simulink model "nms_model"  (Simulink 7.5)
settings: Solver=ode15s  StartTime=0.0  StopTime=60  FixedStep=1e-3  MaxStep=ts_max  RelTol=1e-3  AbsTol=1e-4
InitFcn:
  | nms_model_MechInit
  | nms_model_ControlInit
values from neighbouring files (symbols this model uses):
  c = 0.05    [muscleParams.m]    (also in nms_model_MechInit.m)
  c_jointstop = 0.3 / (pi/180)    (= 17.1887338539)    [muscleParams.m]    (also in nms_model_MechInit.m)
  D12_F = 0.16    [nms_model_MechInit.m]
  D12_S = L_S    (= 0.5)    [nms_model_MechInit.m]
  D12_T = L_T    (= 0.5)    [nms_model_MechInit.m]
  D13_F = 0.20    (= 0.2)    [nms_model_MechInit.m]
  D1G_F = 0.14    [nms_model_MechInit.m]
  D1G_HAT = 0.35    [nms_model_MechInit.m]
  D1G_S = 0.3    [nms_model_MechInit.m]
  D1G_T = 0.3    [nms_model_MechInit.m]
  DeltaThRef = 5e-3    (= 0.005)    [nms_model_MechInit.m]
  eref = 0.04    [muscleParams.m]    (also in nms_model_MechInit.m)
  FmaxGAS = 1500    [nms_model_MechInit.m]
  FmaxGLU = 1500    [nms_model_MechInit.m]
  FmaxHAM = 3000    [nms_model_MechInit.m]
  FmaxHFL = 2000    [nms_model_MechInit.m]
  FmaxSOL = 4000    [nms_model_MechInit.m]
  FmaxTA = 800    [nms_model_MechInit.m]
  FmaxVAS = 300    [muscleParams.m]    (also in nms_model_MechInit.m = 6000)
  GainDeltaTheta = 2 /100*180/pi    (= 1.14591559026)    [nms_model_ControlInit.m]
  GainGAS = 1.1/FmaxGAS    [nms_model_ControlInit.m]
  GainGLU = 0.5/FmaxGLU    [nms_model_ControlInit.m]
  GainHAM = 0.65/FmaxHAM    [nms_model_ControlInit.m]
  GainHAMHFL = 4    [nms_model_ControlInit.m]
  GainHFL = 0.5    [nms_model_ControlInit.m]
  GainKneOverExt = 2    [nms_model_ControlInit.m]
  GainSOL = 1.2/FmaxSOL    [nms_model_ControlInit.m]
  GainSOLTA = 0.4/FmaxSOL    [nms_model_ControlInit.m]
  GainTA = 1.1    [nms_model_ControlInit.m]
  GainVAS = 1.2/FmaxVAS    [nms_model_ControlInit.m]
  In_F = 0.005    [nms_model_MechInit.m]
  In_HAT = 3    [nms_model_MechInit.m]
  In_S = 0.05    [nms_model_MechInit.m]
  In_T = 0.15    [nms_model_MechInit.m]
  K = 5    [muscleParams.m]    (also in nms_model_MechInit.m)
  k_gx = (2*(m_F+m_S+m_T)+m_HAT)*g/0.1    (= 7848)    [nms_model_MechInit.m]
  k_gy = (2*(m_F+m_S+m_T)+m_HAT)*g/0.01    (= 78480)    [nms_model_MechInit.m]
  k_pressure = m_HAT * 9.81 / DeltaThRef    (= 104967)    [nms_model_MechInit.m]
  K_swing = 0.25    [nms_model_ControlInit.m]
  KneePh23Offset = 170*pi/180    (= 2.96705972839)    [nms_model_ControlInit.m]
  LceOffsetHAM = 0.85    [nms_model_ControlInit.m]
  LceOffsetHFL = 0.65    [nms_model_ControlInit.m]
  LceOffsetTA = 1-0.5*w    [nms_model_ControlInit.m]
  LongDelay = 0.020    (= 0.02)    [nms_model_ControlInit.m]
  loptGAS = 0.05    [nms_model_MechInit.m]
  loptGLU = 0.11    [nms_model_MechInit.m]
  loptHAM = 0.10    (= 0.1)    [nms_model_MechInit.m]
  loptHFL = 0.11    [nms_model_MechInit.m]
  loptSOL = 0.04    [nms_model_MechInit.m]
  loptTA = 0.06    [nms_model_MechInit.m]
  loptVAS = 0.13    [muscleParams.m]    (also in nms_model_MechInit.m = 0.08)
  lslackGAS = 0.40    (= 0.4)    [nms_model_MechInit.m]
  lslackGLU = 0.13    [nms_model_MechInit.m]
  lslackHAM = 0.31    [nms_model_MechInit.m]
  lslackHFL = 0.10    (= 0.1)    [nms_model_MechInit.m]
  lslackSOL = 0.26    [nms_model_MechInit.m]
  lslackTA = 0.24    [nms_model_MechInit.m]
  lslackVAS = 0.23    [muscleParams.m]    (also in nms_model_MechInit.m)
  m_F = 1.25    [nms_model_MechInit.m]
  m_HAT = 53.5    [nms_model_MechInit.m]
  m_S = 3.5    [nms_model_MechInit.m]
  m_T = 8.5    [nms_model_MechInit.m]
  MidDelay = 0.010    (= 0.01)    [nms_model_ControlInit.m]
  mu_slide = 0.8    [nms_model_MechInit.m]
  mu_stick = 0.9    [nms_model_MechInit.m]
  N = 1.5    [muscleParams.m]    (also in nms_model_MechInit.m)
  phi12_LowLimit = 70*pi/180    (= 1.2217304764)    [nms_model_MechInit.m]
  phi12_UpLimit = 180*pi/180    (= 3.14159265359)    [muscleParams.m]    (also in nms_model_MechInit.m = 2.26892802759)
  phi23_UpLimit = 159*pi/180    (= 2.77507351067)    [muscleParams.m]    (also in nms_model_MechInit.m = 3.05432619099)
  phi34_UpLimit = 230*pi/180    (= 4.01425727959)    [nms_model_MechInit.m]
  phimaxGASa = 110*pi/180    (= 1.91986217719)    [nms_model_MechInit.m]
  phimaxGASk = 140*pi/180    (= 2.44346095279)    [nms_model_MechInit.m]
  phimaxHAMk = 180*pi/180    (= 3.14159265359)    [nms_model_MechInit.m]
  phimaxSOL = 110*pi/180    (= 1.91986217719)    [nms_model_MechInit.m]
  phimaxTA = 80*pi/180    (= 1.3962634016)    [nms_model_MechInit.m]
  phimaxVAS = 90*pi/180    (= 1.57079632679)    [muscleParams.m]    (also in nms_model_MechInit.m = 2.87979326579)
  phirefGASa = 80*pi/180    (= 1.3962634016)    [nms_model_MechInit.m]
  phirefGASk = 165*pi/180    (= 2.87979326579)    [nms_model_MechInit.m]
  phirefGLU = 150*pi/180    (= 2.61799387799)    [nms_model_MechInit.m]
  phirefHAMh = 155*pi/180    (= 2.70526034059)    [nms_model_MechInit.m]
  phirefHAMk = 180*pi/180    (= 3.14159265359)    [nms_model_MechInit.m]
  phirefHFL = 180*pi/180    (= 3.14159265359)    [nms_model_MechInit.m]
  phirefSOL = 80*pi/180    (= 1.3962634016)    [nms_model_MechInit.m]
  phirefTA = 110*pi/180    (= 1.91986217719)    [nms_model_MechInit.m]
  phirefVAS = 60*pi/180    (= 1.0471975512)    [muscleParams.m]    (also in nms_model_MechInit.m = 2.18166156499)
  PosGainGG = 1/(30*pi/180)    (= 1.9098593171)    [nms_model_ControlInit.m]
  PreStimGAS = 0.01    [nms_model_ControlInit.m]
  PreStimGG = 0.05    [nms_model_ControlInit.m]
  PreStimGLU = 0.01    [nms_model_ControlInit.m]
  PreStimHAM = 0.01    [nms_model_ControlInit.m]
  PreStimHFL = 0.01    [nms_model_ControlInit.m]
  PreStimSOL = 0.01    [nms_model_ControlInit.m]
  PreStimTA = 0.01    [nms_model_ControlInit.m]
  PreStimVAS = 0.08    [nms_model_ControlInit.m]
  rGASa = 0.05    [nms_model_MechInit.m]
  rGASk = 0.05    [nms_model_MechInit.m]
  rGLU = 0.10    (= 0.1)    [nms_model_MechInit.m]
  rHAMh = 0.08    [nms_model_MechInit.m]
  rHAMk = 0.05    [nms_model_MechInit.m]
  rHFL = 0.10    (= 0.1)    [nms_model_MechInit.m]
  rhoGASa = 0.7    [nms_model_MechInit.m]
  rhoGASk = 0.7    [nms_model_MechInit.m]
  rhoGLU = 0.5    [nms_model_MechInit.m]
  rhoHAMh = 0.7    [nms_model_MechInit.m]
  rhoHAMk = 0.7    [nms_model_MechInit.m]
  rhoHFL = 0.5    [nms_model_MechInit.m]
  rhoSOL = 0.5    [nms_model_MechInit.m]
  rhoTA = 0.7    [nms_model_MechInit.m]
  rhoVAS = 3    [muscleParams.m]    (also in nms_model_MechInit.m = 0.7)
  rSOL = 0.05    [nms_model_MechInit.m]
  rTA = 0.04    [nms_model_MechInit.m]
  rVAS = 0.03    [muscleParams.m]    (also in nms_model_MechInit.m = 0.06)
  s = orProblemSendCommand(['LoadIKFastSolver robot Translation3D'],probid)    [init.m]
  ShortDelay = 0.005    [nms_model_ControlInit.m]
  SpeedGainGG = 0.2    [nms_model_ControlInit.m]
  tau = 0.01    [muscleParams.m]    (also in nms_model_MechInit.m)
  Theta0 = 6*pi/180    (= 0.10471975512)    [nms_model_ControlInit.m]
  ThPos = 4/5    (= 0.8)    [nms_model_MechInit.m]
  v_gx_max = 0.03    [nms_model_MechInit.m]
  v_gy_max = 0.03    [nms_model_MechInit.m]
  ... (+11 more)
undefined symbols (not defined in the file or in its folder): sgn
libraries: mblibv1 x60, simulink x22, simulink_extras x20
(part 9 of 9)

== system nms_model/Body Mechanics Layer/Left Ball Contact/Ground Friction Model/X-Axis Kinetic Friction Model ==
  note: Kinetic Friction Model
  note: Footpoint Determiner
  note: Sliding Limit Detector
  pos [m] : Inport  OutDataType=sfix(16)  OutScaling=2^0
  vel [m/s] : Inport  Port=2  OutDataType=sfix(16)  OutScaling=2^0
  F_Normal [N] : Inport  Port=3  OutDataType=sfix(16)  OutScaling=2^0
  Enable : EnablePort  StatesWhenEnabling=reset  ZeroCross=off
  Abs : Abs
  Constant : Constant  Value=vLimit  OutDataType=sfix(16)  OutScaling=2^0
  FixPt Relational Operator : RelationalOperator  Operator=>  LogicOutDataTypeMode=boolean  OutDataTypeStr=boolean  ZeroCross=off
  Memory : Memory
  Negative : simulink/Logic and Bit Operations/Compare To Zero  SystemSampleTime=-1  relop=<  LogicOutDataTypeMode=boolean
  Product : Product  OutDataType=sfix(16)  OutScaling=2^0  RndMeth=Zero
  Sign1 : Signum
  Sum : Sum  Inputs=|+-  OutDataType=sfix(16)  OutScaling=2^0
  reverse : Gain  Gain=-1  ParameterDataType=sfix(16)  ParameterScaling=2^0  OutDataType=sfix(16)  OutScaling=2^0
  sliding friction coefficient : Gain  Gain=mu_slide  ParameterDataType=sfix(16)  ParameterScaling=2^0  OutDataType=sfix(16)  OutScaling=2^0
  posFP [m] : Outport  OutDataType=sfix(16)  OutScaling=2^0  InitialOutput=0
      settings: AttributesFormatString=initial = '%<InitialOutput>'\nwhen disabled = '%<OutputWhenDisabled>'
  Stiction! : Outport  Port=2  OutDataType=sfix(16)  OutScaling=2^0  OutputWhenDisabled=reset  InitialOutput=0
      settings: AttributesFormatString=initial = '%<InitialOutput>'\nwhen disabled = '%<OutputWhenDisabled>'
  F_Slide [N] : Outport  Port=3  OutDataType=sfix(16)  OutScaling=2^0  OutputWhenDisabled=reset  InitialOutput=0
      settings: AttributesFormatString=initial = '%<InitialOutput>'\nwhen disabled = '%<OutputWhenDisabled>'
  wires:
  reverse/1 -> Product/1
  F_Normal [N]/1 -> sliding friction coefficient/1
  vel [m/s]/1 -> Sign1/1, Abs/1
  pos [m]/1 -> posFP [m]/1
  Product/1 -> F_Slide [N]/1
  sliding friction coefficient/1 -> Product/2
  Sign1/1 -> reverse/1
  FixPt Relational Operator/1 -> Stiction!/1
  Memory/1 -> FixPt Relational Operator/2
  Negative/1 -> FixPt Relational Operator/1, Memory/1
  Abs/1 -> Sum/1
  Sum/1 -> Negative/1
  Constant/1 -> Sum/2

== system nms_model/Body Mechanics Layer/Left Ball Contact/Ground Friction Model/X-Axis Static Friction Model ==
  note: Stiction Limit Detector
  note: Static Friction Model
  note: Zero multiplication prevents
      | horizontal friction model from
      | oscillating between static and kinetic
      | friction when the vertical force is zero but
      | the ground level is not yet reached
      | in the upward motion
  F_Normal [N] : Inport  OutDataType=sfix(16)  OutScaling=2^0
  pos [m] : Inport  Port=2  OutDataType=sfix(16)  OutScaling=2^0
  vel [m/s] : Inport  Port=3  OutDataType=sfix(16)  OutScaling=2^0
  posFP [m] : Inport  Port=4  OutDataType=sfix(16)  OutScaling=2^0
  Enable : EnablePort  StatesWhenEnabling=reset  ZeroCross=off
  Abs : Abs
  Abs. : Abs
  Check Vertical Friction : Product  OutDataType=sfix(16)  OutScaling=2^0  RndMeth=Zero
  FixPt Relational Operator : RelationalOperator  Operator=>  LogicOutDataTypeMode=boolean  OutDataTypeStr=boolean  ZeroCross=off
  Gain3 : Gain  Gain=k_gx  ParameterDataType=sfix(16)  ParameterScaling=2^0  OutDataType=sfix(16)  OutScaling=2^0
  Gain4 : Gain  Gain=1/v_gx_max  ParameterDataType=sfix(16)  ParameterScaling=2^0  OutDataType=sfix(16)  OutScaling=2^0
  Memory : Memory
  Mux1 : Mux  Inputs=2
  Positive : simulink/Logic and Bit Operations/Compare To Zero  SystemSampleTime=-1  relop=>  LogicOutDataTypeMode=boolean
  Positive1 : simulink/Logic and Bit Operations/Compare To Zero  SystemSampleTime=-1  relop=>  LogicOutDataTypeMode=boolean
  Sum : Sum  Inputs=-+  OutDataType=sfix(16)  OutScaling=2^0
  Sum2 : Sum  Inputs=-+|  OutDataType=sfix(16)  OutScaling=2^0
  X-Axis Stiction Force : Fcn  Expr=-u(1) * (1+sgn(u(1))*u(2))
  stiction limit force : Gain  Gain=mu_stick  ParameterDataType=sfix(16)  ParameterScaling=2^0  OutDataType=sfix(16)  OutScaling=2^0
  F_Stick [N] : Outport  OutDataType=sfix(16)  OutScaling=2^0  OutputWhenDisabled=reset  InitialOutput=0
      settings: AttributesFormatString=when disabled: %<OutputWhenDisabled>\ninitial: %<InitialOutput>
  Sliding! : Outport  Port=2  OutDataType=sfix(16)  OutScaling=2^0  OutputWhenDisabled=reset  InitialOutput=0
      settings: AttributesFormatString=when disabled: %<OutputWhenDisabled>\ninitial: %<InitialOutput>
  wires:
  F_Normal [N]/1 -> stiction limit force/1, Positive1/1
  Sum2/1 -> Gain3/1  "dx"
  pos [m]/1 -> Sum2/2
  posFP [m]/1 -> Sum2/1
  vel [m/s]/1 -> Gain4/1
  Sum/1 -> Positive/1
  Memory/1 -> FixPt Relational Operator/2
  Positive/1 -> FixPt Relational Operator/1, Memory/1
  Abs./1 -> Sum/2
  Mux1/1 -> X-Axis Stiction Force/1
  Gain3/1 -> Mux1/1
  Gain4/1 -> Mux1/2
  FixPt Relational Operator/1 -> Sliding!/1
  Abs/1 -> Sum/1
  stiction limit force/1 -> Abs/1
  X-Axis Stiction Force/1 -> Check Vertical Friction/1
  Positive1/1 -> Check Vertical Friction/2
  Check Vertical Friction/1 -> F_Stick [N]/1, Abs./1

== system nms_model/Body Mechanics Layer/Left Heel Contact/Ground Friction Model/Friction Switch ==
  note: Static/Kinetic Friction Switch
  Slide! : Inport  OutDataType=sfix(16)  OutScaling=2^0
  Stick! : Inport  Port=2  OutDataType=sfix(16)  OutScaling=2^0
  Memory : Memory
  S-R Flip-Flop : simulink_extras/Flip Flops/S-R Flip-Flop  SystemSampleTime=-1  initial_condition=1
  Terminator : Terminator
  Stiction : Outport  OutDataType=sfix(16)  OutScaling=2^0
  wires:
  Memory/1 -> Stiction/1
  Slide!/1 -> S-R Flip-Flop/2
  Stick!/1 -> S-R Flip-Flop/1
  S-R Flip-Flop/2 -> Terminator/1
  S-R Flip-Flop/1 -> Memory/1

== system nms_model/Body Mechanics Layer/Left Heel Contact/Ground Friction Model/X-Axis Kinetic Friction Model ==
  note: Sliding Limit Detector
  note: Footpoint Determiner
  note: Kinetic Friction Model
  pos [m] : Inport  OutDataType=sfix(16)  OutScaling=2^0
  vel [m/s] : Inport  Port=2  OutDataType=sfix(16)  OutScaling=2^0
  F_Normal [N] : Inport  Port=3  OutDataType=sfix(16)  OutScaling=2^0
  Enable : EnablePort  StatesWhenEnabling=reset  ZeroCross=off
  Abs : Abs
  Constant : Constant  Value=vLimit  OutDataType=sfix(16)  OutScaling=2^0
  FixPt Relational Operator : RelationalOperator  Operator=>  LogicOutDataTypeMode=boolean  OutDataTypeStr=boolean  ZeroCross=off
  Memory : Memory
  Negative : simulink/Logic and Bit Operations/Compare To Zero  SystemSampleTime=-1  relop=<  LogicOutDataTypeMode=boolean
  Product : Product  OutDataType=sfix(16)  OutScaling=2^0  RndMeth=Zero
  Sign1 : Signum
  Sum : Sum  Inputs=|+-  OutDataType=sfix(16)  OutScaling=2^0
  reverse : Gain  Gain=-1  ParameterDataType=sfix(16)  ParameterScaling=2^0  OutDataType=sfix(16)  OutScaling=2^0
  sliding friction coefficient : Gain  Gain=mu_slide  ParameterDataType=sfix(16)  ParameterScaling=2^0  OutDataType=sfix(16)  OutScaling=2^0
  posFP [m] : Outport  OutDataType=sfix(16)  OutScaling=2^0  InitialOutput=0
      settings: AttributesFormatString=initial = '%<InitialOutput>'\nwhen disabled = '%<OutputWhenDisabled>'
  Stiction! : Outport  Port=2  OutDataType=sfix(16)  OutScaling=2^0  OutputWhenDisabled=reset  InitialOutput=0
      settings: AttributesFormatString=initial = '%<InitialOutput>'\nwhen disabled = '%<OutputWhenDisabled>'
  F_Slide [N] : Outport  Port=3  OutDataType=sfix(16)  OutScaling=2^0  OutputWhenDisabled=reset  InitialOutput=0
      settings: AttributesFormatString=initial = '%<InitialOutput>'\nwhen disabled = '%<OutputWhenDisabled>'
  wires:
  Constant/1 -> Sum/2
  Sum/1 -> Negative/1
  Abs/1 -> Sum/1
  Negative/1 -> Memory/1, FixPt Relational Operator/1
  Memory/1 -> FixPt Relational Operator/2
  FixPt Relational Operator/1 -> Stiction!/1
  Sign1/1 -> reverse/1
  sliding friction coefficient/1 -> Product/2
  Product/1 -> F_Slide [N]/1
  pos [m]/1 -> posFP [m]/1
  vel [m/s]/1 -> Abs/1, Sign1/1
  F_Normal [N]/1 -> sliding friction coefficient/1
  reverse/1 -> Product/1

== system nms_model/Body Mechanics Layer/Left Heel Contact/Ground Friction Model/X-Axis Static Friction Model ==
  note: Static Friction Model
  note: Stiction Limit Detector
  note: Zero multiplication prevents
      | horizontal friction model from
      | oscillating between static and kinetic
      | friction when the vertical force is zero but
      | the ground level is not yet reached
      | in the upward motion
  F_Normal [N] : Inport  OutDataType=sfix(16)  OutScaling=2^0
  pos [m] : Inport  Port=2  OutDataType=sfix(16)  OutScaling=2^0
  vel [m/s] : Inport  Port=3  OutDataType=sfix(16)  OutScaling=2^0
  posFP [m] : Inport  Port=4  OutDataType=sfix(16)  OutScaling=2^0
  Enable : EnablePort  StatesWhenEnabling=reset  ZeroCross=off
  Abs : Abs
  Abs. : Abs
  Check Vertical Friction : Product  OutDataType=sfix(16)  OutScaling=2^0  RndMeth=Zero
  FixPt Relational Operator : RelationalOperator  Operator=>  LogicOutDataTypeMode=boolean  OutDataTypeStr=boolean  ZeroCross=off
  Gain3 : Gain  Gain=k_gx  ParameterDataType=sfix(16)  ParameterScaling=2^0  OutDataType=sfix(16)  OutScaling=2^0
  Gain4 : Gain  Gain=1/v_gx_max  ParameterDataType=sfix(16)  ParameterScaling=2^0  OutDataType=sfix(16)  OutScaling=2^0
  Memory : Memory
  Mux1 : Mux  Inputs=2
  Positive : simulink/Logic and Bit Operations/Compare To Zero  SystemSampleTime=-1  relop=>  LogicOutDataTypeMode=boolean
  Positive1 : simulink/Logic and Bit Operations/Compare To Zero  SystemSampleTime=-1  relop=>  LogicOutDataTypeMode=boolean
  Sum : Sum  Inputs=-+  OutDataType=sfix(16)  OutScaling=2^0
  Sum2 : Sum  Inputs=-+|  OutDataType=sfix(16)  OutScaling=2^0
  X-Axis Stiction Force : Fcn  Expr=-u(1) * (1+sgn(u(1))*u(2))
  stiction limit force : Gain  Gain=mu_stick  ParameterDataType=sfix(16)  ParameterScaling=2^0  OutDataType=sfix(16)  OutScaling=2^0
  F_Stick [N] : Outport  OutDataType=sfix(16)  OutScaling=2^0  OutputWhenDisabled=reset  InitialOutput=0
      settings: AttributesFormatString=when disabled: %<OutputWhenDisabled>\ninitial: %<InitialOutput>
  Sliding! : Outport  Port=2  OutDataType=sfix(16)  OutScaling=2^0  OutputWhenDisabled=reset  InitialOutput=0
      settings: AttributesFormatString=when disabled: %<OutputWhenDisabled>\ninitial: %<InitialOutput>
  wires:
  F_Normal [N]/1 -> stiction limit force/1, Positive1/1
  Sum2/1 -> Gain3/1  "dx"
  pos [m]/1 -> Sum2/2
  posFP [m]/1 -> Sum2/1
  vel [m/s]/1 -> Gain4/1
  Sum/1 -> Positive/1
  Memory/1 -> FixPt Relational Operator/2
  Positive/1 -> FixPt Relational Operator/1, Memory/1
  Abs./1 -> Sum/2
  Mux1/1 -> X-Axis Stiction Force/1
  Gain3/1 -> Mux1/1
  Gain4/1 -> Mux1/2
  FixPt Relational Operator/1 -> Sliding!/1
  Abs/1 -> Sum/1
  stiction limit force/1 -> Abs/1
  X-Axis Stiction Force/1 -> Check Vertical Friction/1
  Positive1/1 -> Check Vertical Friction/2
  Check Vertical Friction/1 -> F_Stick [N]/1, Abs./1

== system nms_model/Body Mechanics Layer/Right Ball Contact/Ground Friction Model/Friction Switch ==
  note: Static/Kinetic Friction Switch
  Slide! : Inport  OutDataType=sfix(16)  OutScaling=2^0
  Stick! : Inport  Port=2  OutDataType=sfix(16)  OutScaling=2^0
  Memory : Memory
  S-R Flip-Flop : simulink_extras/Flip Flops/S-R Flip-Flop  SystemSampleTime=-1  initial_condition=1
  Terminator : Terminator
  Stiction : Outport  OutDataType=sfix(16)  OutScaling=2^0
  wires:
  S-R Flip-Flop/1 -> Memory/1
  S-R Flip-Flop/2 -> Terminator/1
  Stick!/1 -> S-R Flip-Flop/1
  Slide!/1 -> S-R Flip-Flop/2
  Memory/1 -> Stiction/1

== system nms_model/Body Mechanics Layer/Right Ball Contact/Ground Friction Model/X-Axis Kinetic Friction Model ==
  note: Kinetic Friction Model
  note: Footpoint Determiner
  note: Sliding Limit Detector
  pos [m] : Inport  OutDataType=sfix(16)  OutScaling=2^0
  vel [m/s] : Inport  Port=2  OutDataType=sfix(16)  OutScaling=2^0
  F_Normal [N] : Inport  Port=3  OutDataType=sfix(16)  OutScaling=2^0
  Enable : EnablePort  StatesWhenEnabling=reset  ZeroCross=off
  Abs : Abs
  Constant : Constant  Value=vLimit  OutDataType=sfix(16)  OutScaling=2^0
  FixPt Relational Operator : RelationalOperator  Operator=>  LogicOutDataTypeMode=boolean  OutDataTypeStr=boolean  ZeroCross=off
  Memory : Memory
  Negative : simulink/Logic and Bit Operations/Compare To Zero  SystemSampleTime=-1  relop=<  LogicOutDataTypeMode=boolean
  Product : Product  OutDataType=sfix(16)  OutScaling=2^0  RndMeth=Zero
  Sign1 : Signum
  Sum : Sum  Inputs=|+-  OutDataType=sfix(16)  OutScaling=2^0
  reverse : Gain  Gain=-1  ParameterDataType=sfix(16)  ParameterScaling=2^0  OutDataType=sfix(16)  OutScaling=2^0
  sliding friction coefficient : Gain  Gain=mu_slide  ParameterDataType=sfix(16)  ParameterScaling=2^0  OutDataType=sfix(16)  OutScaling=2^0
  posFP [m] : Outport  OutDataType=sfix(16)  OutScaling=2^0  InitialOutput=0
      settings: AttributesFormatString=initial = '%<InitialOutput>'\nwhen disabled = '%<OutputWhenDisabled>'
  Stiction! : Outport  Port=2  OutDataType=sfix(16)  OutScaling=2^0  OutputWhenDisabled=reset  InitialOutput=0
      settings: AttributesFormatString=initial = '%<InitialOutput>'\nwhen disabled = '%<OutputWhenDisabled>'
  F_Slide [N] : Outport  Port=3  OutDataType=sfix(16)  OutScaling=2^0  OutputWhenDisabled=reset  InitialOutput=0
      settings: AttributesFormatString=initial = '%<InitialOutput>'\nwhen disabled = '%<OutputWhenDisabled>'
  wires:
  reverse/1 -> Product/1
  F_Normal [N]/1 -> sliding friction coefficient/1
  vel [m/s]/1 -> Sign1/1, Abs/1
  pos [m]/1 -> posFP [m]/1
  Product/1 -> F_Slide [N]/1
  sliding friction coefficient/1 -> Product/2
  Sign1/1 -> reverse/1
  FixPt Relational Operator/1 -> Stiction!/1
  Memory/1 -> FixPt Relational Operator/2
  Negative/1 -> FixPt Relational Operator/1, Memory/1
  Abs/1 -> Sum/1
  Sum/1 -> Negative/1
  Constant/1 -> Sum/2

== system nms_model/Body Mechanics Layer/Right Ball Contact/Ground Friction Model/X-Axis Static Friction Model ==
  note: Stiction Limit Detector
  note: Static Friction Model
  note: Zero multiplication prevents
      | horizontal friction model from
      | oscillating between static and kinetic
      | friction when the vertical force is zero but
      | the ground level is not yet reached
      | in the upward motion
  F_Normal [N] : Inport  OutDataType=sfix(16)  OutScaling=2^0
  pos [m] : Inport  Port=2  OutDataType=sfix(16)  OutScaling=2^0
  vel [m/s] : Inport  Port=3  OutDataType=sfix(16)  OutScaling=2^0
  posFP [m] : Inport  Port=4  OutDataType=sfix(16)  OutScaling=2^0
  Enable : EnablePort  StatesWhenEnabling=reset  ZeroCross=off
  Abs : Abs
  Abs. : Abs
  Check Vertical Friction : Product  OutDataType=sfix(16)  OutScaling=2^0  RndMeth=Zero
  FixPt Relational Operator : RelationalOperator  Operator=>  LogicOutDataTypeMode=boolean  OutDataTypeStr=boolean  ZeroCross=off
  Gain3 : Gain  Gain=k_gx  ParameterDataType=sfix(16)  ParameterScaling=2^0  OutDataType=sfix(16)  OutScaling=2^0
  Gain4 : Gain  Gain=1/v_gx_max  ParameterDataType=sfix(16)  ParameterScaling=2^0  OutDataType=sfix(16)  OutScaling=2^0
  Memory : Memory
  Mux1 : Mux  Inputs=2
  Positive : simulink/Logic and Bit Operations/Compare To Zero  SystemSampleTime=-1  relop=>  LogicOutDataTypeMode=boolean
  Positive1 : simulink/Logic and Bit Operations/Compare To Zero  SystemSampleTime=-1  relop=>  LogicOutDataTypeMode=boolean
  Sum : Sum  Inputs=-+  OutDataType=sfix(16)  OutScaling=2^0
  Sum2 : Sum  Inputs=-+|  OutDataType=sfix(16)  OutScaling=2^0
  X-Axis Stiction Force : Fcn  Expr=-u(1) * (1+sgn(u(1))*u(2))
  stiction limit force : Gain  Gain=mu_stick  ParameterDataType=sfix(16)  ParameterScaling=2^0  OutDataType=sfix(16)  OutScaling=2^0
  F_Stick [N] : Outport  OutDataType=sfix(16)  OutScaling=2^0  OutputWhenDisabled=reset  InitialOutput=0
      settings: AttributesFormatString=when disabled: %<OutputWhenDisabled>\ninitial: %<InitialOutput>
  Sliding! : Outport  Port=2  OutDataType=sfix(16)  OutScaling=2^0  OutputWhenDisabled=reset  InitialOutput=0
      settings: AttributesFormatString=when disabled: %<OutputWhenDisabled>\ninitial: %<InitialOutput>
  wires:
  F_Normal [N]/1 -> stiction limit force/1, Positive1/1
  Sum2/1 -> Gain3/1  "dx"
  pos [m]/1 -> Sum2/2
  posFP [m]/1 -> Sum2/1
  vel [m/s]/1 -> Gain4/1
  Sum/1 -> Positive/1
  Memory/1 -> FixPt Relational Operator/2
  Positive/1 -> FixPt Relational Operator/1, Memory/1
  Abs./1 -> Sum/2
  Mux1/1 -> X-Axis Stiction Force/1
  Gain3/1 -> Mux1/1
  Gain4/1 -> Mux1/2
  FixPt Relational Operator/1 -> Sliding!/1
  Abs/1 -> Sum/1
  stiction limit force/1 -> Abs/1
  X-Axis Stiction Force/1 -> Check Vertical Friction/1
  Positive1/1 -> Check Vertical Friction/2
  Check Vertical Friction/1 -> F_Stick [N]/1, Abs./1

== system nms_model/Body Mechanics Layer/Right Heel Contact/Ground Friction Model/Friction Switch ==
  note: Static/Kinetic Friction Switch
  Slide! : Inport  OutDataType=sfix(16)  OutScaling=2^0
  Stick! : Inport  Port=2  OutDataType=sfix(16)  OutScaling=2^0
  Memory : Memory
  S-R Flip-Flop : simulink_extras/Flip Flops/S-R Flip-Flop  SystemSampleTime=-1  initial_condition=1
  Terminator : Terminator
  Stiction : Outport  OutDataType=sfix(16)  OutScaling=2^0
  wires:
  Memory/1 -> Stiction/1
  Slide!/1 -> S-R Flip-Flop/2
  Stick!/1 -> S-R Flip-Flop/1
  S-R Flip-Flop/2 -> Terminator/1
  S-R Flip-Flop/1 -> Memory/1

== system nms_model/Body Mechanics Layer/Right Heel Contact/Ground Friction Model/X-Axis Kinetic Friction Model ==
  note: Sliding Limit Detector
  note: Footpoint Determiner
  note: Kinetic Friction Model
  pos [m] : Inport  OutDataType=sfix(16)  OutScaling=2^0
  vel [m/s] : Inport  Port=2  OutDataType=sfix(16)  OutScaling=2^0
  F_Normal [N] : Inport  Port=3  OutDataType=sfix(16)  OutScaling=2^0
  Enable : EnablePort  StatesWhenEnabling=reset  ZeroCross=off
  Abs : Abs
  Constant : Constant  Value=vLimit  OutDataType=sfix(16)  OutScaling=2^0
  FixPt Relational Operator : RelationalOperator  Operator=>  LogicOutDataTypeMode=boolean  OutDataTypeStr=boolean  ZeroCross=off
  Memory : Memory
  Negative : simulink/Logic and Bit Operations/Compare To Zero  SystemSampleTime=-1  relop=<  LogicOutDataTypeMode=boolean
  Product : Product  OutDataType=sfix(16)  OutScaling=2^0  RndMeth=Zero
  Sign1 : Signum
  Sum : Sum  Inputs=|+-  OutDataType=sfix(16)  OutScaling=2^0
  reverse : Gain  Gain=-1  ParameterDataType=sfix(16)  ParameterScaling=2^0  OutDataType=sfix(16)  OutScaling=2^0
  sliding friction coefficient : Gain  Gain=mu_slide  ParameterDataType=sfix(16)  ParameterScaling=2^0  OutDataType=sfix(16)  OutScaling=2^0
  posFP [m] : Outport  OutDataType=sfix(16)  OutScaling=2^0  InitialOutput=0
      settings: AttributesFormatString=initial = '%<InitialOutput>'\nwhen disabled = '%<OutputWhenDisabled>'
  Stiction! : Outport  Port=2  OutDataType=sfix(16)  OutScaling=2^0  OutputWhenDisabled=reset  InitialOutput=0
      settings: AttributesFormatString=initial = '%<InitialOutput>'\nwhen disabled = '%<OutputWhenDisabled>'
  F_Slide [N] : Outport  Port=3  OutDataType=sfix(16)  OutScaling=2^0  OutputWhenDisabled=reset  InitialOutput=0
      settings: AttributesFormatString=initial = '%<InitialOutput>'\nwhen disabled = '%<OutputWhenDisabled>'
  wires:
  Constant/1 -> Sum/2
  Sum/1 -> Negative/1
  Abs/1 -> Sum/1
  Negative/1 -> Memory/1, FixPt Relational Operator/1
  Memory/1 -> FixPt Relational Operator/2
  FixPt Relational Operator/1 -> Stiction!/1
  Sign1/1 -> reverse/1
  sliding friction coefficient/1 -> Product/2
  Product/1 -> F_Slide [N]/1
  pos [m]/1 -> posFP [m]/1
  vel [m/s]/1 -> Abs/1, Sign1/1
  F_Normal [N]/1 -> sliding friction coefficient/1
  reverse/1 -> Product/1

== system nms_model/Body Mechanics Layer/Right Heel Contact/Ground Friction Model/X-Axis Static Friction Model ==
  note: Static Friction Model
  note: Stiction Limit Detector
  note: Zero multiplication prevents
      | horizontal friction model from
      | oscillating between static and kinetic
      | friction when the vertical force is zero but
      | the ground level is not yet reached
      | in the upward motion
  F_Normal [N] : Inport  OutDataType=sfix(16)  OutScaling=2^0
  pos [m] : Inport  Port=2  OutDataType=sfix(16)  OutScaling=2^0
  vel [m/s] : Inport  Port=3  OutDataType=sfix(16)  OutScaling=2^0
  posFP [m] : Inport  Port=4  OutDataType=sfix(16)  OutScaling=2^0
  Enable : EnablePort  StatesWhenEnabling=reset  ZeroCross=off
  Abs : Abs
  Abs. : Abs
  Check Vertical Friction : Product  OutDataType=sfix(16)  OutScaling=2^0  RndMeth=Zero
  FixPt Relational Operator : RelationalOperator  Operator=>  LogicOutDataTypeMode=boolean  OutDataTypeStr=boolean  ZeroCross=off
  Gain3 : Gain  Gain=k_gx  ParameterDataType=sfix(16)  ParameterScaling=2^0  OutDataType=sfix(16)  OutScaling=2^0
  Gain4 : Gain  Gain=1/v_gx_max  ParameterDataType=sfix(16)  ParameterScaling=2^0  OutDataType=sfix(16)  OutScaling=2^0
  Memory : Memory
  Mux1 : Mux  Inputs=2
  Positive : simulink/Logic and Bit Operations/Compare To Zero  SystemSampleTime=-1  relop=>  LogicOutDataTypeMode=boolean
  Positive1 : simulink/Logic and Bit Operations/Compare To Zero  SystemSampleTime=-1  relop=>  LogicOutDataTypeMode=boolean
  Sum : Sum  Inputs=-+  OutDataType=sfix(16)  OutScaling=2^0
  Sum2 : Sum  Inputs=-+|  OutDataType=sfix(16)  OutScaling=2^0
  X-Axis Stiction Force : Fcn  Expr=-u(1) * (1+sgn(u(1))*u(2))
  stiction limit force : Gain  Gain=mu_stick  ParameterDataType=sfix(16)  ParameterScaling=2^0  OutDataType=sfix(16)  OutScaling=2^0
  F_Stick [N] : Outport  OutDataType=sfix(16)  OutScaling=2^0  OutputWhenDisabled=reset  InitialOutput=0
      settings: AttributesFormatString=when disabled: %<OutputWhenDisabled>\ninitial: %<InitialOutput>
  Sliding! : Outport  Port=2  OutDataType=sfix(16)  OutScaling=2^0  OutputWhenDisabled=reset  InitialOutput=0
      settings: AttributesFormatString=when disabled: %<OutputWhenDisabled>\ninitial: %<InitialOutput>
  wires:
  F_Normal [N]/1 -> stiction limit force/1, Positive1/1
  Sum2/1 -> Gain3/1  "dx"
  pos [m]/1 -> Sum2/2
  posFP [m]/1 -> Sum2/1
  vel [m/s]/1 -> Gain4/1
  Sum/1 -> Positive/1
  Memory/1 -> FixPt Relational Operator/2
  Positive/1 -> FixPt Relational Operator/1, Memory/1
  Abs./1 -> Sum/2
  Mux1/1 -> X-Axis Stiction Force/1
  Gain3/1 -> Mux1/1
  Gain4/1 -> Mux1/2
  FixPt Relational Operator/1 -> Sliding!/1
  Abs/1 -> Sum/1
  stiction limit force/1 -> Abs/1
  X-Axis Stiction Force/1 -> Check Vertical Friction/1
  Positive1/1 -> Check Vertical Friction/2
  Check Vertical Friction/1 -> F_Stick [N]/1, Abs./1
